simulink model "FHA_2P4S_OL_Rect_Chirp"  (R2018a)
settings: Solver=VariableStepAuto  StartTime=0.0  StopTime=0.05  MaxStep=1e-5  RelTol=1e-3
values from neighbouring files (symbols this model uses):
  Cp = 13.85e-9    (= 1.385e-08)    [Mutual_inductance_Models_Run.m]
  Cs = 16.36e-9    (= 1.636e-08)    [Mutual_inductance_Models_Run.m]
  fop = 156    [Mutual_inductance_Models_Run.m]
  M = [M11 M12; M12' M22]    [Mutual_inductance_Models_Run.m]
  R = [R11 R12;R12' R22]    [Mutual_inductance_Models_Run.m]
  Vin_peak = 127    [Mutual_inductance_Models_Run.m]
libraries: powerlib x47, powerlib_meascontrol x7, dspsrcs4 x5, commutil2 x2, peSinusoidalMeasurement x2, simulink x1, dspxfrm3 x1, dspstat3 x1
settings Model: Creator=user  LastModifiedBy=user

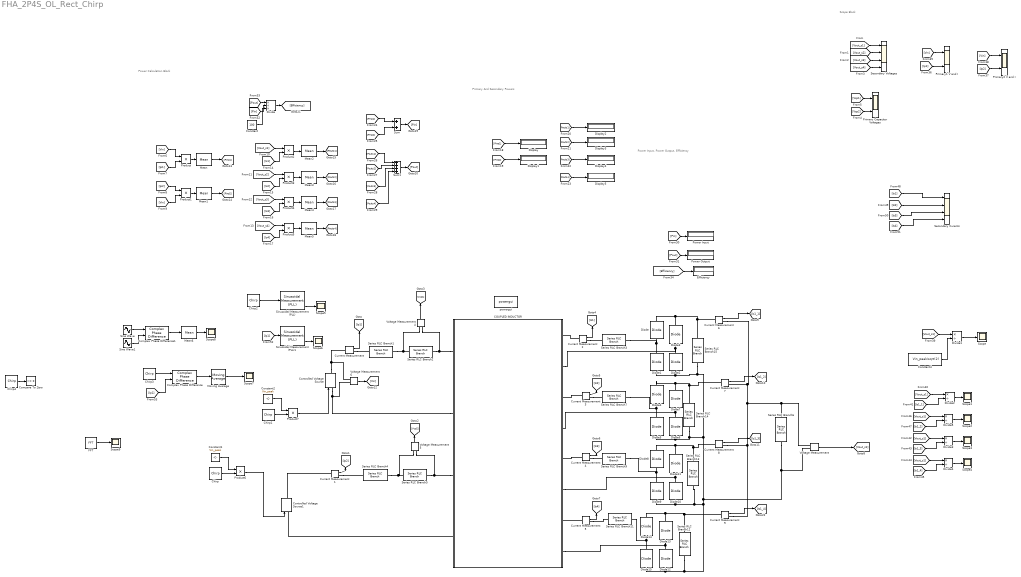
== system FHA_2P4S_OL_Rect_Chirp ==
  note: Scope Block
  note: Primary And Secondary Powers
  note: Power Calculation Block
  note: Power Input,
      | Power Output,
      | Efficiency
  COUPLED INDUCTOR : Subsystem
  Chirp{,1..4} (5 alike) : dspsrcs4/Chirp  sweep=Linear  mode=Unidirectional  f0=1e5  f1=2e5  t1=0.05  Tsweep=1  phase=0  Ts=1e-7  spf=1  datatype=Double  OutputFrames=off
      settings: SourceProductName=DSP System Toolbox
  Compare To Zero : simulink/Logic and Bit Operations/Compare To Zero  relop=<=  OutDataTypeStr=boolean
  Complex Phase Difference : commutil2/Complex Phase Difference
      settings: SourceProductName=Communications System Toolbox  SourceProductBaseCode=CM
  Complex Phase Difference1 : commutil2/Complex Phase Difference
      settings: SourceProductName=Communications System Toolbox  SourceProductBaseCode=CM
  Constant : Constant  Value=100
  Constant1 : Constant  Value=Vin_peak
  Constant2 : Constant  Value=Vin_peak
  Constant4 : Constant  Value=Vin_peak/sqrt(2)
  Controlled Voltage Source : powerlib/Electrical Sources/Controlled Voltage Source  Initialize=on  Source_Type=AC  Amplitude=0  Phase=0  Frequency=0  Measurements=None
  Controlled Voltage Source1 : powerlib/Electrical Sources/Controlled Voltage Source  Initialize=on  Source_Type=AC  Amplitude=0  Phase=0  Frequency=0  Measurements=None
  Current Measurement{,1..9} (10 alike) : powerlib/Measurements/Current Measurement  PhasorSimulation=off  OutputType=Complex  PSBequivalent=0
  Diode{,1..15} (16 alike) : powerlib/Power Electronics/Diode  Ron=0.001  Lon=0  Vf=0.8  IC=0  UseSnubber=0  Rs=inf  Cs=250e-9  Measurements=off
  Display{,1..5} (6 alike) : Display
  Divide : Product  Inputs=*/*
  Divide{1..5} (5 alike) : Product  Inputs=*/
  Efficiency : Display
  FFT : dspxfrm3/FFT  FFTImplementation=Auto  CompMethod=Table lookup  TableOpt=NEW  TableOptActive=Speed  BitRevOrder=on  Normalize=on  InheritFFTLength=on  FFTLength=64  WrapInput=on  roundingMode=Floor  overflowMode=off  firstCoeffDataTypeStr=Inherit: Same word length as input  firstCoeffLastDataTypeStr=Inherit: Same word length as input  outputMin=[]  outputMax=[]
  Mean{,1..5} (6 alike) : powerlib_meascontrol/Measurements/Mean  Freq=fop*1000  Vinit=0  Ts=0
  Mean6 : powerlib_meascontrol/Measurements/Mean  Freq=150000  Vinit=0  Ts=0
  Moving Average : dspstat3/Moving Average  Method=Sliding window  ForgettingFactorPort=off  SpecifyWindowLength=on  WindowLength=600  ForgettingFactor=0.9  SimulateUsing=Code generation
  Power Input : Display
  Power Output : Display
  Primary Capacitor Voltages : Scope  NumInputPorts=2
  Primary1 V and I : Scope  NumInputPorts=2
  Primary2 V and I : Scope  NumInputPorts=2
  Product{,1..7} (8 alike) : Product
  Scope{,1..9} (10 alike) : Scope
  Secondary Curents : Scope  NumInputPorts=4
  Secondary Voltages : Scope  NumInputPorts=4
  Series RLC Branch1 : powerlib/Elements/Series RLC Branch  LConnTagsString=__new0  RConnTagsString=__new0  BranchType=R  Resistance=0.01  Inductance=1e-3  SetiL0=off  InitialCurrent=0  Capacitance=1e-6  Setx0=off  InitialVoltage=0  Measurements=None
  Series RLC Branch{3,7,9,11} (4 alike) : powerlib/Elements/Series RLC Branch  LConnTagsString=__new0  RConnTagsString=__new0  BranchType=C  Resistance=0.01  Inductance=1e-3  SetiL0=off  InitialCurrent=0  Capacitance=Cs  Setx0=off  InitialVoltage=0  Measurements=None
  Series RLC Branch{12..15} (4 alike) : powerlib/Elements/Series RLC Branch  LConnTagsString=__new0  RConnTagsString=__new0  BranchType=C  Resistance=70  Inductance=1e-3  SetiL0=off  InitialCurrent=0  Capacitance=1e-6  Setx0=off  InitialVoltage=0  Measurements=None
  Series RLC Branch2 : powerlib/Elements/Series RLC Branch  LConnTagsString=__new0  RConnTagsString=__new0  BranchType=C  Resistance=0.01  Inductance=1e-3  SetiL0=off  InitialCurrent=0  Capacitance=Cp  Setx0=off  InitialVoltage=0  Measurements=None
  Series RLC Branch4 : powerlib/Elements/Series RLC Branch  LConnTagsString=__new0  RConnTagsString=__new0  BranchType=R  Resistance=0.01  Inductance=1e-3  SetiL0=off  InitialCurrent=0  Capacitance=1e-6  Setx0=off  InitialVoltage=0  Measurements=None
  Series RLC Branch5 : powerlib/Elements/Series RLC Branch  LConnTagsString=__new0  RConnTagsString=__new0  BranchType=C  Resistance=0.01  Inductance=1e-3  SetiL0=off  InitialCurrent=0  Capacitance=Cp  Setx0=off  InitialVoltage=0  Measurements=None
  Series RLC Branch6 : powerlib/Elements/Series RLC Branch  LConnTagsString=__new0  RConnTagsString=__new0  BranchType=R  Resistance=10  Inductance=1e-3  SetiL0=off  InitialCurrent=0  Capacitance=1e-6  Setx0=off  InitialVoltage=0  Measurements=None
  Sine Wave : Sin  Frequency=2*pi*150000  SampleTime=0
  Sine Wave1 : Sin  Frequency=2*pi*150000  Phase=1  SampleTime=0
  Sinusoidal Measurement (PLL) : peSinusoidalMeasurement/Sinusoidal Measurement (PLL)  Ki_PD=1000  Kp_LF=400  Ki_LF=20000  F0=60  Theta0=0  Mag0=1  Ts=-1
  Sinusoidal Measurement (PLL)1 : peSinusoidalMeasurement/Sinusoidal Measurement (PLL)  Ki_PD=1000  Kp_LF=400  Ki_LF=20000  F0=60  Theta0=0  Mag0=1  Ts=-1
  Sum : Sum
  Sum1 : Sum  Inputs=++++
  Voltage Measurement{,4..6} (4 alike) : powerlib/Measurements/Voltage Measurement  PhasorSimulation=off  OutputType=Complex  PSBequivalent=0
  powergui : powerlib/powergui  Priority=1  SimulationMode=Continuous  SampleTime=50e-6  frequency=60  Iterations=50  frequencyindice=0  Pbase=100e6  ErrMax=1e-4  UnitsV=kV  UnitsW=MW  buscounter=0  FunctionMessages=off  echomessages=off  EnableUseOfTLC=off  CurrentSourceSwitches=off  DisableSnubberDevices=off  DisableRonSwitches=off  DisableVfSwitches=off  DisplayEquations=off  SolverType=Tustin/Backward Euler (TBE)  Interpol=off  ExternalGateDelay=off  methode=off  Ts=100  x0status=blocks  SPID=on  SwTol=0  HookPort=off  RestoreLinks=warning  ResistiveCurrentMeasurement=off  Frange=[0:2:500]  Ylog=off  Xlog=on  ShowGrid=off  save=off  variable=ZData  structure=0  ZoomFFT=off  StartTime=0.0  cycles=1  DisplayStyle=1  fundamental=60  FreqAxis=off  MaxFrequency=1000  frequencyindicesteady=1  RmsSteady=1  display=off
  wires:
  Divide/1 -> [Efficiency]
  [Ip1] -> Primary1 V and I/2
  [Efficiency] -> Efficiency/1
  [Pouts4] -> Sum1/4
  [Vin] -> Primary1 V and I/1
  [Vin] -> Primary2 V and I/1
  [Pin] -> Power Input/1
  Mean1/1 -> [Pinp2]
  [Pin] -> Divide/2
  [Pout] -> Divide/1
  [Vout_s2] -> Product3/1
  Constant/1 -> Divide/3
  Current Measurement/1 -> [Ip1]
  [Pouts3] -> Sum1/3
  [Pinp1] -> Sum/1
  [Pout] -> Power Output/1
  [Vout_s3] -> Secondary Voltages/3
  [Vout_s1] -> Product2/1
  Current Measurement4/1 -> [Is3]
  [Pouts2] -> Sum1/2
  Sum1/1 -> [Pout]
  Current Measurement1/1 -> [Ip2]
  [Is2] -> Product3/2
  [Pouts2] -> Display3/1
  [Pouts3] -> Display4/1
  [Pinp2] -> Display1/1
  [Pouts1] -> Display2/1
  [Pinp2] -> Sum/2
  [Vcp1] -> Primary Capacitor Voltages/1
  [Pinp1] -> Display/1
  [Pouts4] -> Display5/1
  Product5/1 -> Mean5/1
  [Vin] -> Product/1
  [Vout_s2] -> Secondary Voltages/2
  Mean/1 -> [Pinp1]
  [Is4] -> Product5/2
  Mean4/1 -> [Pouts3]
  Mean2/1 -> [Pouts1]
  Product2/1 -> Mean2/1
  Product4/1 -> Mean4/1
  [Vcp2] -> Primary Capacitor Voltages/2
  [Vout_s4] -> Product5/1
  [Is1] -> Product2/2
  [Vin] -> Product1/2
  [Vout_s1] -> Secondary Voltages/1
  [Ip1] -> Product/2
  [Pouts1] -> Sum1/1
  Voltage Measurement4/1 -> [Vcp1]
  [Vout_s3] -> Product4/1
  Product7/1 -> Controlled Voltage Source/1
  Current Measurement3/1 -> [Is2]
  Product1/1 -> Mean1/1
  Mean3/1 -> [Pouts2]
  Sum/1 -> [Pin]
  [Ip2] -> Product1/1
  Mean5/1 -> [Pouts4]
  Voltage Measurement/1 -> [Vout_s1]
  [Vout_s4] -> Secondary Voltages/4
  [Ip2] -> Primary2 V and I/2
  [Is3] -> Product4/2
  Current Measurement2/1 -> [Is1]
  Product/1 -> Mean/1
  Voltage Measurement5/1 -> [Vcp2]
  Product3/1 -> Mean3/1
  Current Measurement5/1 -> [Is4]
  Voltage Measurement6/1 -> [Vin]
  Chirp/1 -> Product6/2
  Constant1/1 -> Product6/1
  Product6/1 -> Controlled Voltage Source1/1
  Chirp1/1 -> Product7/2
  Constant2/1 -> Product7/1
  [Vout_s1] -> Divide1/1
  Constant4/1 -> Divide1/2
  Divide1/1 -> Scope/1
  Current Measurement6/1 -> [Is1_1]
  Current Measurement7/1 -> [Is1_2]
  Current Measurement8/1 -> [Is1_3]
  Current Measurement9/1 -> [Is1_4]
  [Vout_s1] -> Divide2/1
  [Is1_1] -> Divide2/2
  [Vout_s1] -> Divide3/1
  [Is1_3] -> Divide3/2
  [Vout_s1] -> Divide4/1
  [Is1_4] -> Divide4/2
  [Vout_s1] -> Divide5/1
  [Is1_2] -> Divide5/2
  Divide5/1 -> Scope2/1
  Divide4/1 -> Scope4/1
  Divide3/1 -> Scope3/1
  Divide2/1 -> Scope1/1
  [Is1] -> Secondary Curents/1
  [Is2] -> Secondary Curents/2
  [Is3] -> Secondary Curents/3
  [Is4] -> Secondary Curents/4
  Chirp2/1 -> Sinusoidal Measurement (PLL)/1
  Sinusoidal Measurement (PLL)/3 -> Scope5/1
  [Ip1] -> Sinusoidal Measurement (PLL)1/1
  Sinusoidal Measurement (PLL)1/3 -> Scope6/1
  Chirp3/1 -> Complex Phase Difference/1
  [Ip1] -> Complex Phase Difference/2
  Complex Phase Difference/1 -> Moving Average/1
  Sine Wave/1 -> Complex Phase Difference1/1
  Sine Wave1/1 -> Complex Phase Difference1/2
  Complex Phase Difference1/1 -> Mean6/1
  Mean6/1 -> Scope8/1
  Moving Average/1 -> Scope7/1
  FFT/1 -> Scope9/1
  Chirp4/1 -> Compare To Zero/1
  connections:
  Diode14/RConn1 -- Current Measurement9/LConn1 -- Series RLC Branch12/LConn1 -- Diode13/RConn1
  Series RLC Branch2/LConn1 -- Series RLC Branch1/LConn1 -- Voltage Measurement4/LConn1
  Series RLC Branch5/LConn1 -- Series RLC Branch4/LConn1 -- Voltage Measurement5/LConn1
  Controlled Voltage Source/RConn1 -- Current Measurement/LConn1 -- Voltage Measurement6/LConn1
  COUPLED INDUCTOR/RConn3 -- Series RLC Branch5/RConn1 -- Voltage Measurement5/LConn2
  COUPLED INDUCTOR/RConn1 -- Series RLC Branch2/RConn1 -- Voltage Measurement4/LConn2
  COUPLED INDUCTOR/RConn2 -- Controlled Voltage Source/LConn1 -- Voltage Measurement6/LConn2
  Current Measurement1/LConn1 -- Controlled Voltage Source1/RConn1
  Current Measurement/RConn1 -- Series RLC Branch1/RConn1
  Current Measurement3/RConn1 -- Series RLC Branch7/LConn1
  Current Measurement4/LConn1 -- COUPLED INDUCTOR/LConn5
  Current Measurement5/RConn1 -- Series RLC Branch11/LConn1
  Current Measurement2/LConn1 -- COUPLED INDUCTOR/LConn1
  Current Measurement5/LConn1 -- COUPLED INDUCTOR/LConn7
  Current Measurement2/RConn1 -- Series RLC Branch3/LConn1
  COUPLED INDUCTOR/RConn4 -- Controlled Voltage Source1/LConn1
  Current Measurement3/LConn1 -- COUPLED INDUCTOR/LConn3
  Current Measurement4/RConn1 -- Series RLC Branch9/LConn1
  Current Measurement1/RConn1 -- Series RLC Branch4/RConn1
  Diode1/RConn1 -- Series RLC Branch3/RConn1 -- Diode/LConn1
  Diode3/LConn1 -- COUPLED INDUCTOR/LConn2 -- Diode2/RConn1
  Diode7/LConn1 -- COUPLED INDUCTOR/LConn4 -- Diode6/RConn1
  Diode5/RConn1 -- Series RLC Branch7/RConn1 -- Diode4/LConn1
  Diode9/RConn1 -- Series RLC Branch9/RConn1 -- Diode8/LConn1
  Diode11/LConn1 -- COUPLED INDUCTOR/LConn6 -- Diode10/RConn1
  Diode6/LConn1 -- Voltage Measurement/LConn2 -- Series RLC Branch6/RConn1 -- Diode9/LConn1 -- Diode10/LConn1 -- Series RLC Branch13/RConn1 -- Diode12/LConn1 -- Diode15/LConn1 -- Series RLC Branch12/RConn1 -- Diode2/LConn1 -- Diode1/LConn1 -- Series RLC Branch15/RConn1 -- Series RLC Branch14/RConn1 -- Diode5/LConn1
  Diode13/LConn1 -- COUPLED INDUCTOR/LConn8 -- Diode12/RConn1
  Diode15/RConn1 -- Series RLC Branch11/RConn1 -- Diode14/LConn1
  Diode/RConn1 -- Current Measurement6/LConn1 -- Series RLC Branch15/LConn1 -- Diode3/RConn1
  Diode4/RConn1 -- Current Measurement7/LConn1 -- Series RLC Branch14/LConn1 -- Diode7/RConn1
  Diode8/RConn1 -- Current Measurement8/LConn1 -- Series RLC Branch13/LConn1 -- Diode11/RConn1
  Series RLC Branch6/LConn1 -- Voltage Measurement/LConn1 -- Current Measurement7/RConn1 -- Current Measurement6/RConn1 -- Current Measurement9/RConn1 -- Current Measurement8/RConn1

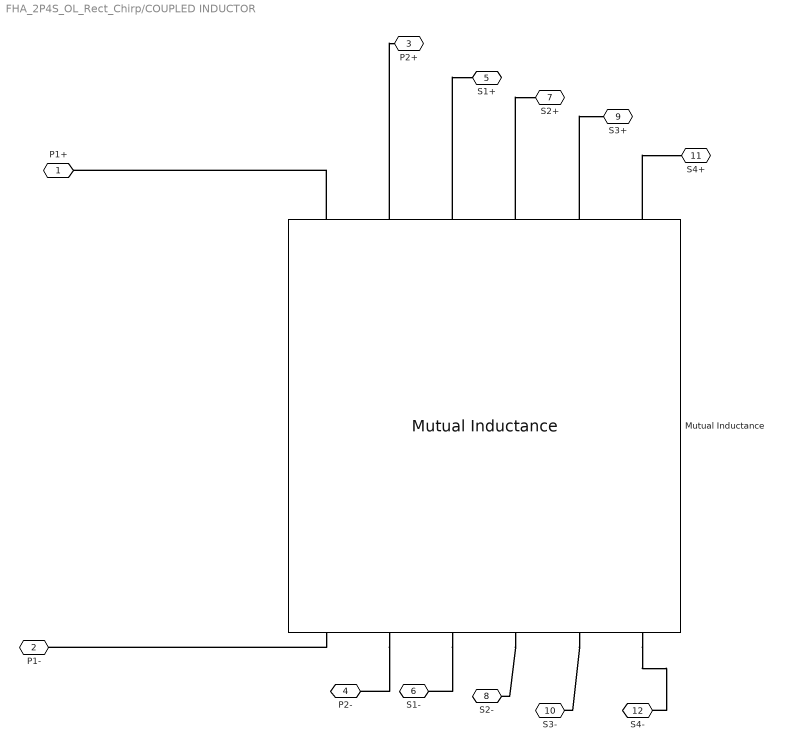
== system FHA_2P4S_OL_Rect_Chirp/COUPLED INDUCTOR ==
  Mutual Inductance : powerlib/Elements/Mutual Inductance  LConnTagsString=a|b|c|L4|L5|L6  RConnTagsString=A|B|C|R4|R5|R6  TypeOfMutual=Generalized mutual inductance  NumberOfWindings=6  SelfImpedance1=[1.1 1.1e-03]  SelfImpedance2=[ 1.1 1.1e-03]  ThreeWindings=on  SelfImpedance3=[ 1.1 1.1e-03]  MutualImpedance=[1.0 1.0e-03]  InductanceMatrix=M * 1e-6  ResistanceMatrix=R*0.001  Measurements=None
      settings: AttributesFormatString=\n  SourceProductName=Simscape Power Systems  SourceProductBaseCode=PS
  P1+ : PMIOPort  Side=Right
  P1- : PMIOPort  Port=2  Side=Right
  P2+ : PMIOPort  Port=3  Side=Right
  P2- : PMIOPort  Port=4  Side=Right
  S1+ : PMIOPort  Port=5  Side=Left
  S1- : PMIOPort  Port=6  Side=Left
  S2+ : PMIOPort  Port=7  Side=Left
  S2- : PMIOPort  Port=8  Side=Left
  S3+ : PMIOPort  Port=9  Side=Left
  S3- : PMIOPort  Port=10  Side=Left
  S4+ : PMIOPort  Port=11  Side=Left
  S4- : PMIOPort  Port=12  Side=Left
  connections:
  Mutual Inductance/LConn2 -- P2-/RConn1
  Mutual Inductance/LConn5 -- S3-/RConn1
  Mutual Inductance/RConn5 -- S3+/RConn1
  Mutual Inductance/RConn4 -- S2+/RConn1
  Mutual Inductance/LConn6 -- S4-/RConn1
  Mutual Inductance/RConn1 -- P1+/RConn1
  Mutual Inductance/LConn1 -- P1-/RConn1
  Mutual Inductance/RConn2 -- P2+/RConn1
  Mutual Inductance/LConn4 -- S2-/RConn1
  Mutual Inductance/LConn3 -- S1-/RConn1
  Mutual Inductance/RConn3 -- S1+/RConn1
  Mutual Inductance/RConn6 -- S4+/RConn1
